simulink model "HW4_Q1_2014a"  (Simulink 10.2)
settings: Solver=ode45  StartTime=0.0  StopTime=10000  FixedStep=2  RelTol=1e-3  EnableMultiTasking=on
libraries: simulink x4
settings Model: Creator=Sudchai Boonto  LastModifiedBy=Benyamin (hamireZ)
settings DataIOCC: LimitDataPoints=on
settings OptimizationCC: ExpressionDepthLimit=2147483647
settings DebuggingCC: SolverPrmCheckMsg=warning  StateNameClashWarn=warning

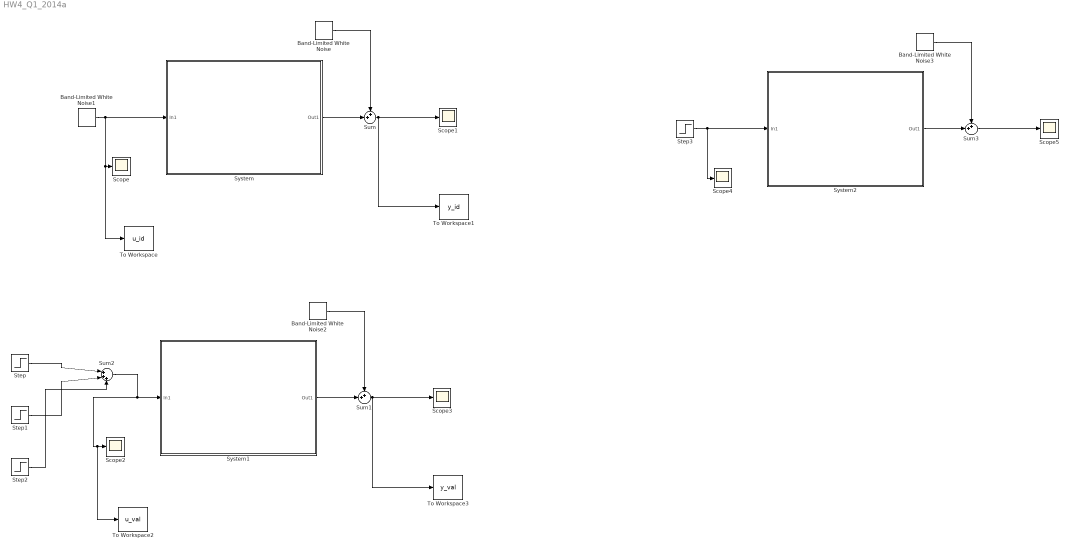
== system HW4_Q1_2014a ==
  Band-Limited White Noise : simulink/Sources/Band-Limited White Noise  Cov=[0.01]  Ts=4.5  seed=[23341]
  Band-Limited White Noise1 : simulink/Sources/Band-Limited White Noise  Cov=[5]  Ts=4.5  seed=[23341]
  Band-Limited White Noise2 : simulink/Sources/Band-Limited White Noise  Cov=[0.01]  Ts=4.5  seed=[23341]
  Band-Limited White Noise3 : simulink/Sources/Band-Limited White Noise  Cov=[0.01]  Ts=2  seed=[23341]
  Scope{,1..5} (6 alike) : Scope
  Step : Step  Time=2000  Before=1  After=0  SampleTime=4.5
  Step1 : Step  Time=3000  After=-2.5  SampleTime=4.5
  Step2 : Step  Time=7000  After=3.5  SampleTime=4.5
  Step3 : Step  Time=10  SampleTime=1
  Sum : Sum  Inputs=++|
  Sum1 : Sum  Inputs=++|
  Sum2 : Sum  Inputs=|+++
  Sum3 : Sum  Inputs=++|
  System : Subsystem  mask(Rotary Dryer){}
      mask help: This is a rotary dryer for sugar beets. The input to the process is the amount of fuel supplied m_dot and the output is the amount of dry matter phi_DM.
      mask Display: image(imread('dryer.jpg'))
  System1 : Subsystem  mask(Rotary Dryer){}
      mask help: This is a rotary dryer for sugar beets. The input to the process is the amount of fuel supplied m_dot and the output is the amount of dry matter phi_DM.
      mask Display: image(imread('dryer.jpg'))
  System2 : Subsystem  mask(Rotary Dryer){}
      mask help: This is a rotary dryer for sugar beets. The input to the process is the amount of fuel supplied m_dot and the output is the amount of dry matter phi_DM.
      mask Display: image(imread('dryer.jpg'))
  To Workspace : ToWorkspace  VariableName=u_id  SampleTime=4.5
      settings: Save2DSignal=2-D array (concatenate along first dimension)
  To Workspace1 : ToWorkspace  VariableName=y_id  SampleTime=4.5
      settings: Save2DSignal=2-D array (concatenate along first dimension)
  To Workspace2 : ToWorkspace  VariableName=u_val  SampleTime=4.5
      settings: Save2DSignal=2-D array (concatenate along first dimension)
  To Workspace3 : ToWorkspace  VariableName=y_val  SampleTime=4.5
      settings: Save2DSignal=2-D array (concatenate along first dimension)
  wires:
  System/1(Out1) -> Sum/2
  Band-Limited White Noise/1 -> Sum/1
  Band-Limited White Noise1/1 -> To Workspace/1, Scope/1, System/1(In1)
  Sum/1 -> To Workspace1/1, Scope1/1
  Sum1/1 -> Scope3/1, To Workspace3/1
  Band-Limited White Noise2/1 -> Sum1/1
  System1/1(Out1) -> Sum1/2
  Step1/1 -> Sum2/2
  Step/1 -> Sum2/1
  Sum2/1 -> System1/1(In1), To Workspace2/1, Scope2/1
  Step2/1 -> Sum2/3
  Sum3/1 -> Scope5/1
  Step3/1 -> System2/1(In1), Scope4/1
  Band-Limited White Noise3/1 -> Sum3/1
  System2/1(Out1) -> Sum3/2

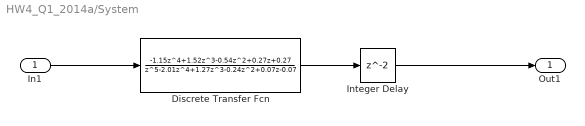
== system HW4_Q1_2014a/System ==
  In1 : Inport
  Discrete Transfer Fcn : DiscreteTransferFcn  Numerator=[-1.15 1.52 -0.54 0.27 0.27]  Denominator="[1  -2.01 1.27 -0.24 0.07 -0.07]"  SampleTime=2
  Integer Delay : Delay
  Out1 : Outport
  wires:
  In1/1 -> Discrete Transfer Fcn/1
  Discrete Transfer Fcn/1 -> Integer Delay/1
  Integer Delay/1 -> Out1/1

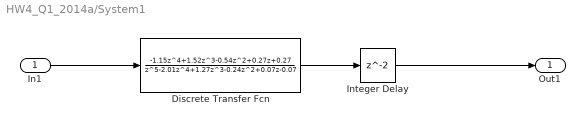
== system HW4_Q1_2014a/System1 ==
  In1 : Inport
  Discrete Transfer Fcn : DiscreteTransferFcn  Numerator=[-1.15 1.52 -0.54 0.27 0.27]  Denominator="[1  -2.01 1.27 -0.24 0.07 -0.07]"  SampleTime=2
  Integer Delay : Delay
  Out1 : Outport
  wires:
  Integer Delay/1 -> Out1/1
  Discrete Transfer Fcn/1 -> Integer Delay/1
  In1/1 -> Discrete Transfer Fcn/1

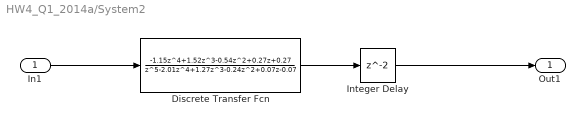
== system HW4_Q1_2014a/System2 ==
  In1 : Inport
  Discrete Transfer Fcn : DiscreteTransferFcn  Numerator=[-1.15 1.52 -0.54 0.27 0.27]  Denominator="[1  -2.01 1.27 -0.24 0.07 -0.07]"  SampleTime=2
  Integer Delay : Delay
  Out1 : Outport
  wires:
  Integer Delay/1 -> Out1/1
  Discrete Transfer Fcn/1 -> Integer Delay/1
  In1/1 -> Discrete Transfer Fcn/1
